simulink model "vgammaRegler"  (R2017a)
settings: Solver=VariableStepAuto  StartTime=0.0  StopTime=10.0  RelTol=1e-3
values from neighbouring files (symbols this model uses):
  h = 1000    [Minv.m]    (also in Roboterdaten.m)
  l_a = 0.14    [Minv.m]    (also in Roboterdaten.m)
  r = 0.1    [Minv.m]    (also in Roboterdaten.m)
undefined symbols (not defined in the file or in its folder): G_mot, la, R_Kipp_Roboter
settings Model: Creator=Timo  LastModifiedBy=Timo

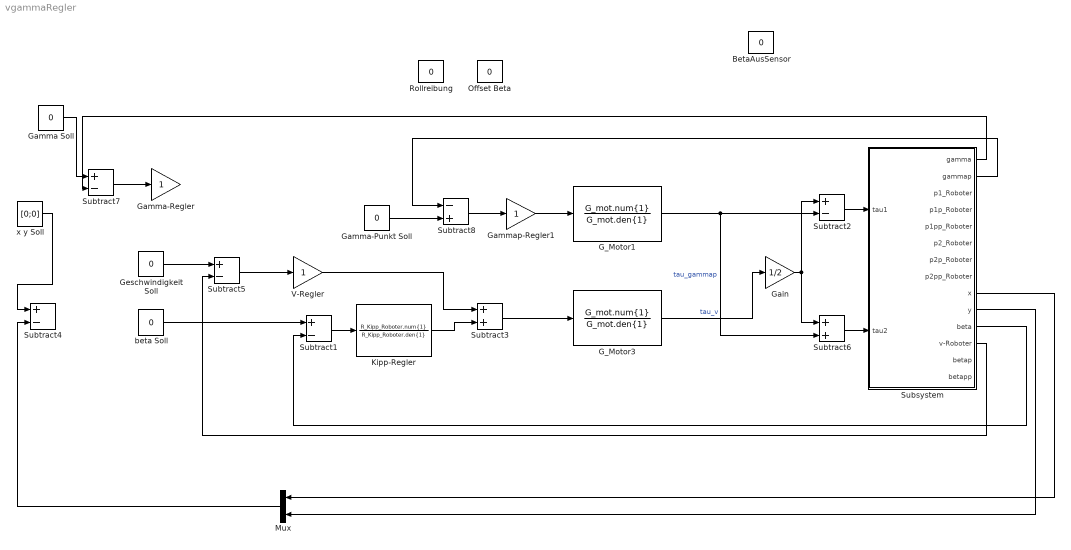
== system vgammaRegler ==
  BetaAusSensor : Constant  Value=0
  G_Motor1 : TransferFcn  Numerator=G_mot.num{1}  Denominator=G_mot.den{1}
  G_Motor3 : TransferFcn  Numerator=G_mot.num{1}  Denominator=G_mot.den{1}
  Gain : Gain  Gain=1/2
  Gamma Soll : Constant  Value=0
  Gamma-Punkt Soll : Constant  Value=0
  Gamma-Regler : Gain
  Gammap-Regler1 : Gain
  Geschwindigkeit Soll : Constant  Value=0
  Kipp-Regler : TransferFcn  Numerator=R_Kipp_Roboter.num{1}  Denominator=R_Kipp_Roboter.den{1}
  Mux : Mux  Inputs=2
  Offset Beta : Constant  Value=0
  Rollreibung : Constant  Value=0
  Subsystem : Subsystem
  Subtract{1..2,4..5,7} (5 alike) : Sum  Inputs=+-
  Subtract3 : Sum
  Subtract6 : Sum
  Subtract8 : Sum  Inputs=-+
  V-Regler : Gain
  beta Soll : Constant  Value=0
  x y Soll : Constant  Value=[0;0]
  wires:
  Subsystem/9(x) -> Mux/1
  Subsystem/10(y) -> Mux/2
  Mux/1 -> Subtract4/2
  x y Soll/1 -> Subtract4/1
  Kipp-Regler/1 -> Subtract3/2
  Subtract1/1 -> Kipp-Regler/1
  beta Soll/1 -> Subtract1/1
  Subsystem/11(beta) -> Subtract1/2
  V-Regler/1 -> Subtract3/1
  Subtract3/1 -> G_Motor3/1
  G_Motor3/1 -> Gain/1  "tau_v"
  Subtract7/1 -> Gamma-Regler/1
  Geschwindigkeit Soll/1 -> Subtract5/1
  Subtract5/1 -> V-Regler/1
  Subsystem/12(v-Roboter) -> Subtract5/2
  Subsystem/1(gamma) -> Subtract7/2
  Gamma Soll/1 -> Subtract7/1
  Gain/1 -> Subtract6/1, Subtract2/1
  Subtract2/1 -> Subsystem/1(tau1)
  Subtract6/1 -> Subsystem/2(tau2)
  Gammap-Regler1/1 -> G_Motor1/1
  Subsystem/2(gammap) -> Subtract8/1
  Subtract8/1 -> Gammap-Regler1/1
  Gamma-Punkt Soll/1 -> Subtract8/2
  G_Motor1/1 -> Subtract2/2, Subtract6/2  "tau_gammap"

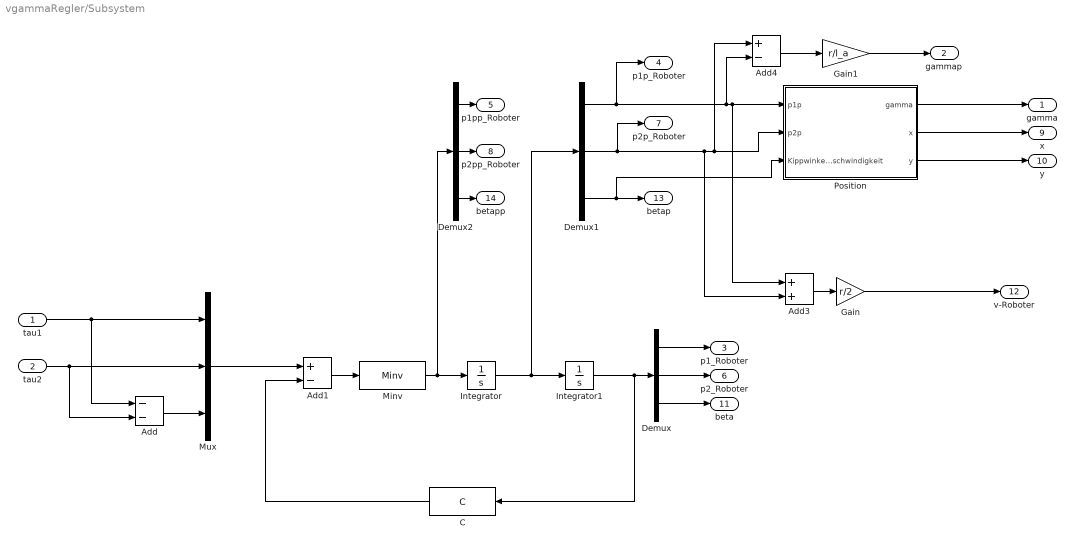
== system vgammaRegler/Subsystem ==
  tau1 : Inport
  tau2 : Inport  Port=2
  Add : Sum  Inputs=--
  Add1 : Sum  Inputs=+-
  Add3 : Sum
  Add4 : Sum  Inputs=+-
  C : MATLABFcn  MATLABFcn=C  OutputDimensions=3
  Demux : Demux  Outputs=3
  Demux1 : Demux  Outputs=3
  Demux2 : Demux  Outputs=3
  Gain : Gain  Gain=r/2
  Gain1 : Gain  Gain=r/l_a
  Integrator : Integrator
  Integrator1 : Integrator
  Minv : MATLABFcn  MATLABFcn=Minv  OutputDimensions=3
  Mux : Mux  Inputs=3
  Position : Subsystem
  gamma : Outport
  gammap : Outport  Port=2
  p1_Roboter : Outport  Port=3
  p1p_Roboter : Outport  Port=4
  p1pp_Roboter : Outport  Port=5
  p2_Roboter : Outport  Port=6
  p2p_Roboter : Outport  Port=7
  p2pp_Roboter : Outport  Port=8
  x : Outport  Port=9
  y : Outport  Port=10
  beta : Outport  Port=11
  v-Roboter : Outport  Port=12
  betap : Outport  Port=13
  betapp : Outport  Port=14
  wires:
  tau1/1 -> Mux/1, Add/1
  tau2/1 -> Mux/2, Add/2
  Add/1 -> Mux/3
  Mux/1 -> Add1/1
  Integrator/1 -> Demux1/1, Integrator1/1
  Add1/1 -> Minv/1
  Integrator1/1 -> C/1, Demux/1
  Demux/1 -> p1_Roboter/1
  Demux/2 -> p2_Roboter/1
  Demux/3 -> beta/1
  Demux1/3 -> Position/3(Kippwinkelgeschwindigkeit), betap/1
  Demux1/2 -> p2p_Roboter/1, Add4/1, Position/2(p2p), Add3/2
  Demux1/1 -> p1p_Roboter/1, Add4/2, Position/1(p1p), Add3/1
  C/1 -> Add1/2
  Demux2/2 -> p2pp_Roboter/1
  Demux2/1 -> p1pp_Roboter/1
  Demux2/3 -> betapp/1
  Minv/1 -> Demux2/1, Integrator/1
  Position/1(gamma) -> gamma/1
  Position/2(x) -> x/1
  Position/3(y) -> y/1
  Add3/1 -> Gain/1
  Add4/1 -> Gain1/1
  Gain1/1 -> gammap/1
  Gain/1 -> v-Roboter/1

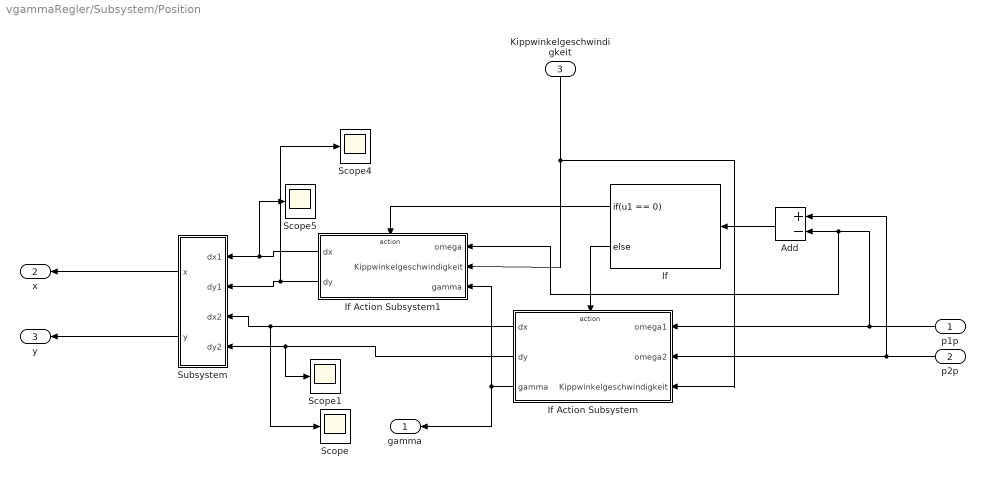
== system vgammaRegler/Subsystem/Position ==
  p1p : Inport
  p2p : Inport  Port=2
  Kippwinkelgeschwindigkeit : Inport  Port=3
  Add : Sum  Inputs=+-
  If : If  IfExpression=u1 == 0
  If Action Subsystem : Subsystem  TreatAsAtomicUnit=on
  If Action Subsystem1 : Subsystem  TreatAsAtomicUnit=on
  Scope{,1,4..5} (4 alike) : Scope
  Subsystem : Subsystem
  gamma : Outport
  x : Outport  Port=2
  y : Outport  Port=3
  wires:
  If Action Subsystem/2(dy) -> Scope1/1, Subsystem/4(dy2)
  If Action Subsystem1/2(dy) -> Scope4/1, Subsystem/2(dy1)
  If Action Subsystem1/1(dx) -> Scope5/1, Subsystem/1(dx1)
  If/1 -> If Action Subsystem1/Action
  Kippwinkelgeschwindigkeit/1 -> If Action Subsystem/3(Kippwinkelgeschwindigkeit), If Action Subsystem1/2(Kippwinkelgeschwindigkeit)
  Subsystem/2(y) -> y/1
  p1p/1 -> If Action Subsystem1/1(omega), Add/2, If Action Subsystem/1(omega1)
  If Action Subsystem/1(dx) -> Scope/1, Subsystem/3(dx2)
  If Action Subsystem/3(gamma) -> gamma/1, If Action Subsystem1/3(gamma)
  If/2 -> If Action Subsystem/Action
  p2p/1 -> Add/1, If Action Subsystem/2(omega2)
  Add/1 -> If/1
  Subsystem/1(x) -> x/1

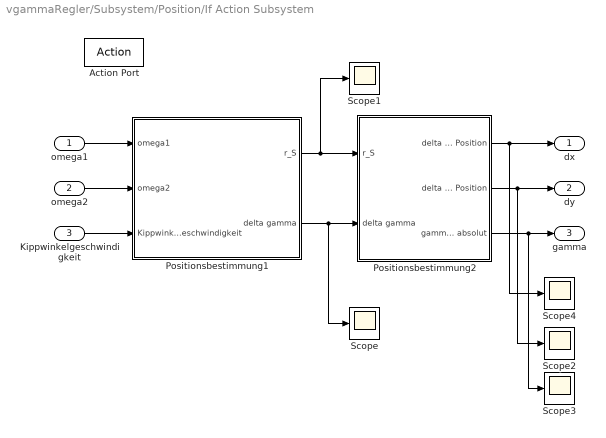
== system vgammaRegler/Subsystem/Position/If Action Subsystem ==
  omega1 : Inport
  omega2 : Inport  Port=2
  Kippwinkelgeschwindigkeit : Inport  Port=3
  Action Port : ActionPort
  Positionsbestimmung1 : Subsystem
  Positionsbestimmung2 : Subsystem
  Scope{,1..4} (5 alike) : Scope
  dx : Outport
  dy : Outport  Port=2
  gamma : Outport  Port=3
  wires:
  Positionsbestimmung1/1(r_S) -> Scope1/1, Positionsbestimmung2/1(r_S)
  Positionsbestimmung1/2(delta gamma) -> Scope/1, Positionsbestimmung2/2(delta gamma)
  omega1/1 -> Positionsbestimmung1/1(omega1)
  omega2/1 -> Positionsbestimmung1/2(omega2)
  Kippwinkelgeschwindigkeit/1 -> Positionsbestimmung1/3(Kippwinkelgeschwindigkeit)
  Positionsbestimmung2/1(delta x Position) -> Scope4/1, dx/1
  Positionsbestimmung2/3(gamma absolut) -> Scope3/1, gamma/1
  Positionsbestimmung2/2(delta y Position) -> Scope2/1, dy/1

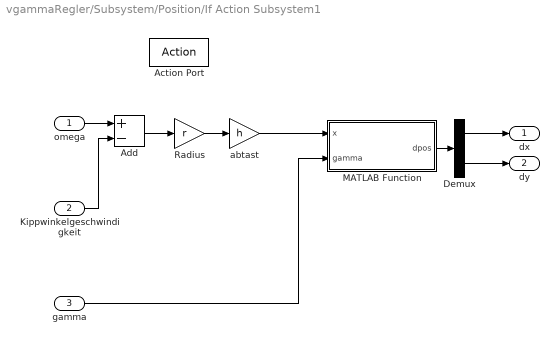
== system vgammaRegler/Subsystem/Position/If Action Subsystem1 ==
  omega : Inport
  Kippwinkelgeschwindigkeit : Inport  Port=2
  gamma : Inport  Port=3
  Action Port : ActionPort
  Add : Sum  Inputs=+-
  Demux : Demux  Outputs=2
  MATLAB Function : MATLAB Function  TreatAsAtomicUnit=on
  Radius : Gain  Gain=r
  abtast : Gain  Gain=h
  dx : Outport
  dy : Outport  Port=2
  wires:
  gamma/1 -> MATLAB Function/2(gamma)
  Radius/1 -> abtast/1
  abtast/1 -> MATLAB Function/1(x)
  MATLAB Function/1(dpos) -> Demux/1
  Demux/1 -> dx/1
  Demux/2 -> dy/1
  Add/1 -> Radius/1
  omega/1 -> Add/1
  Kippwinkelgeschwindigkeit/1 -> Add/2

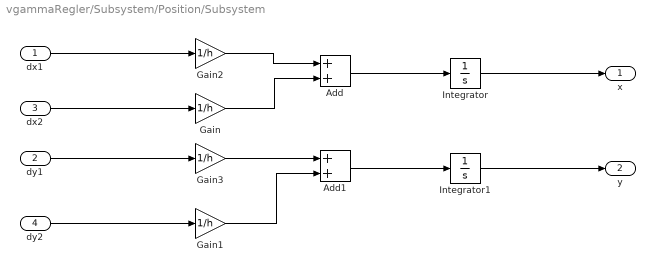
== system vgammaRegler/Subsystem/Position/Subsystem ==
  dx1 : Inport
  dy1 : Inport  Port=2
  dx2 : Inport  Port=3
  dy2 : Inport  Port=4
  Add : Sum
  Add1 : Sum
  Gain{,1..3} (4 alike) : Gain  Gain=1/h
  Integrator : Integrator
  Integrator1 : Integrator
  x : Outport
  y : Outport  Port=2
  wires:
  dy1/1 -> Gain3/1
  dx1/1 -> Gain2/1
  dx2/1 -> Gain/1
  dy2/1 -> Gain1/1
  Gain2/1 -> Add/1
  Gain/1 -> Add/2
  Gain3/1 -> Add1/1
  Gain1/1 -> Add1/2
  Add1/1 -> Integrator1/1
  Add/1 -> Integrator/1
  Integrator/1 -> x/1
  Integrator1/1 -> y/1

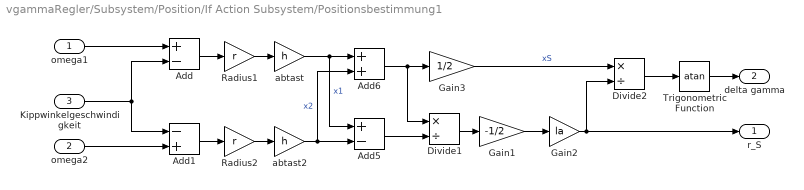
== system vgammaRegler/Subsystem/Position/If Action Subsystem/Positionsbestimmung1 ==
  omega1 : Inport
  omega2 : Inport  Port=2
  Kippwinkelgeschwindigkeit : Inport  Port=3
  Add : Sum  Inputs=+-
  Add1 : Sum  Inputs=-+
  Add5 : Sum  Inputs=+-
  Add6 : Sum
  Divide1 : Product  Inputs=*/
  Divide2 : Product  Inputs=*/
  Gain1 : Gain  Gain=-1/2
  Gain2 : Gain  Gain=la
  Gain3 : Gain  Gain=1/2
  Radius1 : Gain  Gain=r
  Radius2 : Gain  Gain=r
  Trigonometric Function : Trigonometry  Operator=atan
  abtast : Gain  Gain=h
  abtast2 : Gain  Gain=h
  r_S : Outport
  delta gamma : Outport  Port=2
  wires:
  omega1/1 -> Add/1
  Kippwinkelgeschwindigkeit/1 -> Add/2, Add1/1
  omega2/1 -> Add1/2
  Add/1 -> Radius1/1
  Add1/1 -> Radius2/1
  Radius1/1 -> abtast/1
  Radius2/1 -> abtast2/1
  abtast2/1 -> Add5/2, Add6/2  "x2"
  abtast/1 -> Add6/1, Add5/1  "x1"
  Add6/1 -> Gain3/1, Divide1/1
  Add5/1 -> Divide1/2
  Divide1/1 -> Gain1/1
  Gain1/1 -> Gain2/1
  Gain2/1 -> r_S/1, Divide2/2
  Gain3/1 -> Divide2/1  "xS"
  Trigonometric Function/1 -> delta gamma/1
  Divide2/1 -> Trigonometric Function/1

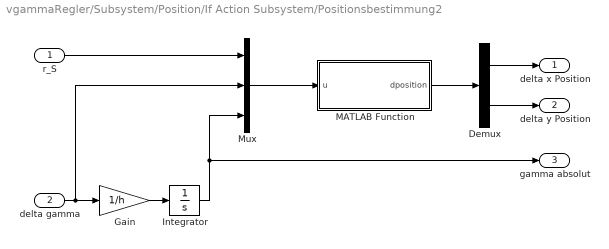
== system vgammaRegler/Subsystem/Position/If Action Subsystem/Positionsbestimmung2 ==
  r_S : Inport
  delta gamma : Inport  Port=2
  Demux : Demux  Outputs=2
  Gain : Gain  Gain=1/h
  Integrator : Integrator
  MATLAB Function : MATLAB Function  TreatAsAtomicUnit=on
  Mux : Mux  Inputs=3
  delta x Position : Outport
  delta y Position : Outport  Port=2
  gamma absolut : Outport  Port=3
  wires:
  delta gamma/1 -> Gain/1, Mux/2
  Mux/1 -> MATLAB Function/1(u)
  r_S/1 -> Mux/1
  MATLAB Function/1(dposition) -> Demux/1
  Demux/1 -> delta x Position/1
  Demux/2 -> delta y Position/1
  Integrator/1 -> gamma absolut/1, Mux/3
  Gain/1 -> Integrator/1

== matlab function vgammaRegler/Subsystem/Position/If Action Subsystem1/MATLAB Function ==
  data: x input; dpos output; gamma input
function dpos = fcn(x, gamma)


dpos = [x*cos(gamma); x*sin(gamma)];

== matlab function vgammaRegler/Subsystem/Position/If Action Subsystem/Positionsbestimmung2/MATLAB Function ==
  data: u input; dposition output
function dposition  = fcn(u)

r = u(1);
dgamma = u(2);
gamma = u(3);

dposition = [r*(sin(gamma+dgamma)-sin(gamma)); r*(cos(gamma)-cos(gamma+dgamma))];
